simulink model "truck_cabin_sim"  (R2025b)
settings: Solver=FixedStepAuto  StartTime=0.0  StopTime=1000  RelTol=1e-3
values from neighbouring files (symbols this model uses):
  Cth = 50000    [parameters.m]
  HSI_RH_bp = [      0      7.5      17.5      27.5      32.5      37.5      47.5      52.5      72.5      92.5 ]    [HSI_LUT_Setup.m]
  HSI_T_bp = 20:39    [HSI_LUT_Setup.m]
  HSI_Table = 255 * ones(      length(HSI_T_bp),      length(HSI_RH_bp))    [HSI_LUT_Setup.m]
  LowTemp = 20    [HSI_LUT_Setup.m]    (also in hsi_parameters.m = 4)
  Qcool = 3000    [parameters.m]
  RH_initial = 60    [parameters.m]
  T_initial = 25    [parameters.m]
  T_sensor_sigma = 0.2    [parameters.m]
  Ts = 1    [parameters.m]
  UA = 100    [parameters.m]
libraries: simulink x1
settings Model: SnapshotBufferSize=1000  SnapshotInterval=1000  Creator=Admin  LastModifiedBy=Admin
settings OptimizationCC: DefaultParameterBehavior=Inlined  UseDivisionForNetSlopeComputation=on  GainParamInheritBuiltInType=on  UseFloatMulNetSlope=on  InlineInvariantSignals=on  PassReuseOutputArgsAs=Individual arguments  ZeroExternalMemoryAtStartup=off  ZeroInternalMemoryAtStartup=off  NoFixptDivByZeroProtection=on  EfficientFloat2IntCast=on  LifeSpan=1  OptimizeBlockOrder=speed  DifferentSizesBufferReuse=on  EfficientTunableParamExpr=on
settings DebuggingCC: ParameterTunabilityLossMsg=error
settings HardwareCC: ProdLongLongMode=on
settings SFSimCC: MATLABDynamicMemAlloc=off
settings RTWCC: SystemTargetFile=ert.tlc  GenCodeOnly=on  TemplateMakefile=ert_default_tmf  Description=Embedded Coder
settings CodeAppCC: ForceParamTrailComments=on  IgnoreCustomStorageClasses=off  OperatorAnnotations=on  SimulinkDataObjDesc=on  SFDataObjDesc=on  CustomSymbolStrGlobalVar=rt$N$M  CustomSymbolStrType=$N$M  CustomSymbolStrFcn=$N$M$F  CustomSymbolStrMacro=$N$M  InsertBlockDesc=on
settings ERTTargetCC: ERTCustomFileTemplate=example_file_process.tlc  ERTFilePackagingFormat=CompactWithDataFile  TargetLangStandard=C99 (ISO)  GenerateSampleERTMain=on  IncludeMdlTerminateFcn=off  CombineSignalStateStructs=on  SupportComplex=off  SupportContinuousTime=on  SupportNonInlinedSFcns=on

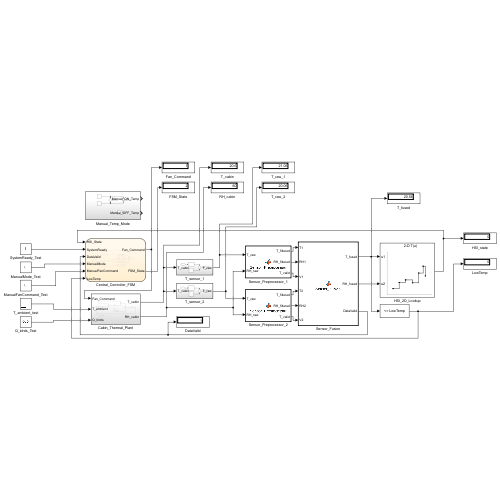
[thumbnail: Simulink's stored preview of the top-level diagram]
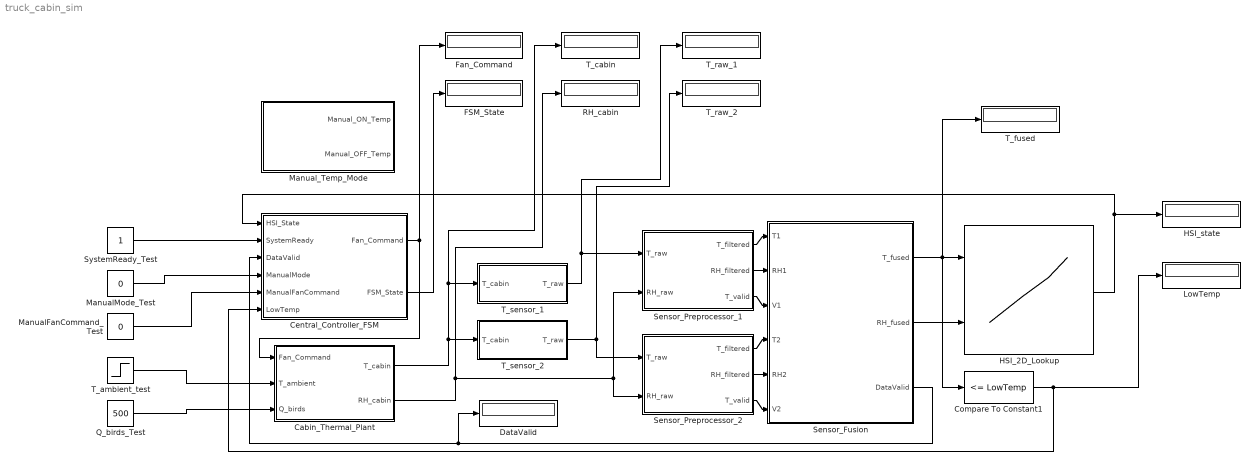
== system truck_cabin_sim ==
  Cabin_Thermal_Plant : Subsystem
  Central_Controller_FSM : Stateflow chart  TreatAsAtomicUnit=on
  Compare To Constant1 : simulink/Logic and Bit Operations/Compare To Constant  relop=<=  const=LowTemp  OutDataTypeStr=boolean
  DataValid : Display
  FSM_State : Display
  Fan_Command : Display
  HSI_2D_Lookup : Lookup_n-D  BreakpointsForDimension1=HSI_T_bp  BreakpointsForDimension2=HSI_RH_bp  Table=HSI_Table  InterpMethod=Flat  InternalRulePriority=Speed  RndMeth=Simplest
      settings: InputPortMap=u0,u1
  HSI_state : Display
  LowTemp : Display
  ManualFanCommand_Test : Constant  Value=0
  ManualMode_Test : Constant  Value=0
  Manual_Temp_Mode : Subsystem
  Q_birds_Test : Constant  Value=500
  RH_cabin : Display
  Sensor_Fusion : MATLAB Function  TreatAsAtomicUnit=on  SystemSampleTime=1
  Sensor_Preprocessor_1 : MATLAB Function  TreatAsAtomicUnit=on  SystemSampleTime=1
  Sensor_Preprocessor_2 : MATLAB Function  TreatAsAtomicUnit=on  SystemSampleTime=1
  SystemReady_Test : Constant
  T_ambient_test : Step  Time=60  Before=20  After=35  SampleTime=Ts
  T_cabin : Display
  T_fused : Display
  T_raw_1 : Display
  T_raw_2 : Display
  T_sensor_1 : Subsystem
  T_sensor_2 : Subsystem
  wires:
  T_ambient_test/1 -> Cabin_Thermal_Plant/2(T_ambient)
  Sensor_Preprocessor_2/2(RH_filtered) -> Sensor_Fusion/5(RH2)
  Sensor_Preprocessor_1/1(T_filtered) -> Sensor_Fusion/1(T1)
  Sensor_Preprocessor_1/2(RH_filtered) -> Sensor_Fusion/2(RH1)
  Sensor_Preprocessor_1/3(T_valid) -> Sensor_Fusion/3(V1)
  Sensor_Preprocessor_2/1(T_filtered) -> Sensor_Fusion/4(T2)
  Sensor_Preprocessor_2/3(T_valid) -> Sensor_Fusion/6(V2)
  Cabin_Thermal_Plant/1(T_cabin) -> T_cabin/1, T_sensor_1/1(T_cabin), T_sensor_2/1(T_cabin)
  T_sensor_1/1(T_raw) -> Sensor_Preprocessor_1/1(T_raw), T_raw_1/1
  T_sensor_2/1(T_raw) -> T_raw_2/1, Sensor_Preprocessor_2/1(T_raw)
  Cabin_Thermal_Plant/2(RH_cabin) -> RH_cabin/1, Sensor_Preprocessor_2/2(RH_raw), Sensor_Preprocessor_1/2(RH_raw)
  Central_Controller_FSM/1(Fan_Command) -> Cabin_Thermal_Plant/1(Fan_Command), Fan_Command/1
  SystemReady_Test/1 -> Central_Controller_FSM/2(SystemReady)
  ManualFanCommand_Test/1 -> Central_Controller_FSM/5(ManualFanCommand)
  ManualMode_Test/1 -> Central_Controller_FSM/4(ManualMode)
  Q_birds_Test/1 -> Cabin_Thermal_Plant/3(Q_birds)
  Central_Controller_FSM/2(FSM_State) -> FSM_State/1
  Sensor_Fusion/3(DataValid) -> Central_Controller_FSM/3(DataValid), DataValid/1
  Sensor_Fusion/2(RH_fused) -> HSI_2D_Lookup/2
  HSI_2D_Lookup/1 -> HSI_state/1, Central_Controller_FSM/1(HSI_State)
  Sensor_Fusion/1(T_fused) -> HSI_2D_Lookup/1, Compare To Constant1/1, T_fused/1
  Compare To Constant1/1 -> LowTemp/1, Central_Controller_FSM/6(LowTemp)

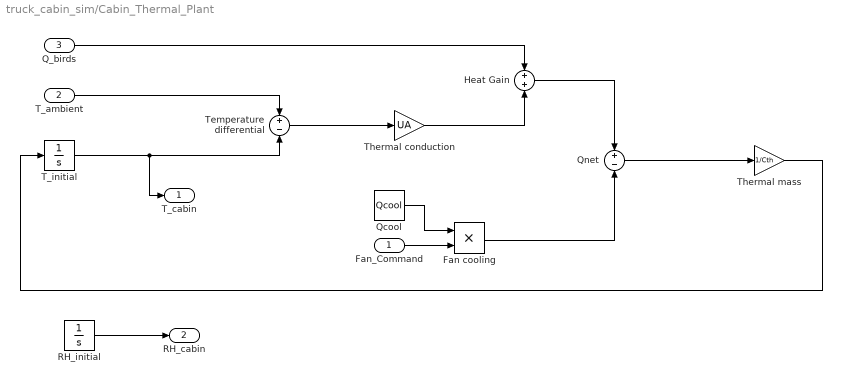
== system truck_cabin_sim/Cabin_Thermal_Plant ==
  Fan_Command : Inport
  T_ambient : Inport  Port=2
  Q_birds : Inport  Port=3
  Fan cooling : Product
  Heat Gain : Sum
  Qcool : Constant  Value=Qcool
  Qnet : Sum  Inputs=+-
  RH_initial : Integrator  InitialCondition=RH_initial
  T_initial : Integrator  InitialCondition=T_initial
  Temperature differential : Sum  Inputs=+-
  Thermal conduction : Gain  Gain=UA
  Thermal mass : Gain  Gain=1/Cth
  T_cabin : Outport
  RH_cabin : Outport  Port=2
  wires:
  T_ambient/1 -> Temperature differential/1
  Temperature differential/1 -> Thermal conduction/1
  Q_birds/1 -> Heat Gain/1
  Thermal conduction/1 -> Heat Gain/2
  Qcool/1 -> Fan cooling/1
  Fan_Command/1 -> Fan cooling/2
  Fan cooling/1 -> Qnet/2
  Heat Gain/1 -> Qnet/1
  Qnet/1 -> Thermal mass/1
  T_initial/1 -> T_cabin/1, Temperature differential/2
  Thermal mass/1 -> T_initial/1
  RH_initial/1 -> RH_cabin/1

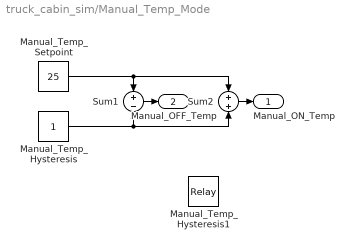
== system truck_cabin_sim/Manual_Temp_Mode ==
  Manual_Temp_Hysteresis : Constant
  Manual_Temp_Hysteresis1 : Relay
  Manual_Temp_Setpoint : Constant  Value=25
  Sum1 : Sum  Inputs=+-
  Sum2 : Sum
  Manual_ON_Temp : Outport
  Manual_OFF_Temp : Outport  Port=2
  wires:
  Manual_Temp_Setpoint/1 -> Sum2/1, Sum1/1
  Manual_Temp_Hysteresis/1 -> Sum2/2, Sum1/2
  Sum2/1 -> Manual_ON_Temp/1
  Sum1/1 -> Manual_OFF_Temp/1

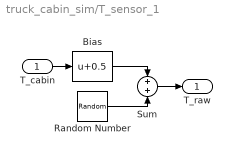
== system truck_cabin_sim/T_sensor_1 ==
  T_cabin : Inport
  Bias : Bias  Bias=0.5  SaturateOnIntegerOverflow=off
  Random Number : RandomNumber  Variance=T_sensor_sigma^2  SampleTime=Ts
  Sum : Sum
  T_raw : Outport
  wires:
  Bias/1 -> Sum/1
  Random Number/1 -> Sum/2
  T_cabin/1 -> Bias/1
  Sum/1 -> T_raw/1

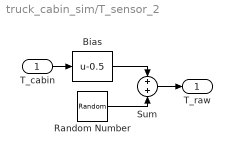
== system truck_cabin_sim/T_sensor_2 ==
  T_cabin : Inport
  Bias : Bias  Bias=-0.5  SaturateOnIntegerOverflow=off
  Random Number : RandomNumber  Variance=T_sensor_sigma^2  SampleTime=Ts
  Sum : Sum
  T_raw : Outport
  wires:
  Bias/1 -> Sum/1
  Random Number/1 -> Sum/2
  T_cabin/1 -> Bias/1
  Sum/1 -> T_raw/1

== matlab function truck_cabin_sim/Sensor_Preprocessor_1 ==
  data: T_raw input; T_filtered output; RH_raw input; RH_filtered output; T_valid output
function [T_filtered, RH_filtered, T_valid] = ...
    Sensor_Preprocessor(T_raw, RH_raw)

persistent T_buffer
persistent RH_buffer
persistent PreviousAcceptedT

if isempty(T_buffer)

    T_buffer = T_raw * ones(1,5);
    RH_buffer = RH_raw * ones(1,5);

    PreviousAcceptedT = T_raw;

end

% ---------------------------------------------------------
% 1. Reject excessive temperature rate
% ---------------------------------------------------------

TempRate = abs(T_raw - PreviousAcceptedT);

if TempRate > 3

    T_valid = false;

    AcceptedT = PreviousAcceptedT;

else

    T_valid = true;

    AcceptedT = T_raw;

    PreviousAcceptedT = T_raw;

end

% ---------------------------------------------------------
% 2. Shift temperature window
% ---------------------------------------------------------

T_buffer(1) = T_buffer(2);
T_buffer(2) = T_buffer(3);
T_buffer(3) = T_buffer(4);
T_buffer(4) = T_buffer(5);
T_buffer(5) = AcceptedT;

% ---------------------------------------------------------
% 3. Shift RH window
% ---------------------------------------------------------

RH_buffer(1) = RH_buffer(2);
RH_buffer(2) = RH_buffer(3);
RH_buffer(3) = RH_buffer(4);
RH_buffer(4) = RH_buffer(5);
RH_buffer(5) = RH_raw;

% ---------------------------------------------------------
% 4. Median
% ---------------------------------------------------------

SortedT = sort(T_buffer);
SortedRH = sort(RH_buffer);

T_filtered = SortedT(3);
RH_filtered = SortedRH(3);

end

== matlab function truck_cabin_sim/Sensor_Preprocessor_2 ==
  data: T_raw input; T_filtered output; RH_raw input; RH_filtered output; T_valid output
function [T_filtered, RH_filtered, T_valid] = ...
    Sensor_Preprocessor(T_raw, RH_raw)

persistent T_buffer
persistent RH_buffer
persistent PreviousAcceptedT

if isempty(T_buffer)

    T_buffer = T_raw * ones(1,5);
    RH_buffer = RH_raw * ones(1,5);

    PreviousAcceptedT = T_raw;

end

% ---------------------------------------------------------
% 1. Reject excessive temperature rate
% ---------------------------------------------------------

TempRate = abs(T_raw - PreviousAcceptedT);

if TempRate > 3

    T_valid = false;

    AcceptedT = PreviousAcceptedT;

else

    T_valid = true;

    AcceptedT = T_raw;

    PreviousAcceptedT = T_raw;

end

% ---------------------------------------------------------
% 2. Shift temperature window
% ---------------------------------------------------------

T_buffer(1) = T_buffer(2);
T_buffer(2) = T_buffer(3);
T_buffer(3) = T_buffer(4);
T_buffer(4) = T_buffer(5);
T_buffer(5) = AcceptedT;

% ---------------------------------------------------------
% 3. Shift RH window
% ---------------------------------------------------------

RH_buffer(1) = RH_buffer(2);
RH_buffer(2) = RH_buffer(3);
RH_buffer(3) = RH_buffer(4);
RH_buffer(4) = RH_buffer(5);
RH_buffer(5) = RH_raw;

% ---------------------------------------------------------
% 4. Median
% ---------------------------------------------------------

SortedT = sort(T_buffer);
SortedRH = sort(RH_buffer);

T_filtered = SortedT(3);
RH_filtered = SortedRH(3);

end

== matlab function truck_cabin_sim/Sensor_Fusion ==
  data: T1 input; T_fused output; RH1 input; V1 input; T2 input; RH2 input; V2 input; RH_fused output; DataValid output
function [T_fused, RH_fused, DataValid] = ...
    Sensor_Fusion(T1, RH1, V1, T2, RH2, V2)

w1 = 0.5;
w2 = 0.5;

sumT = 0;
sumRH = 0;
sumW = 0;

if V1
    sumT = sumT + w1*T1;
    sumRH = sumRH + w1*RH1;
    sumW = sumW + w1;
end

if V2
    sumT = sumT + w2*T2;
    sumRH = sumRH + w2*RH2;
    sumW = sumW + w2;
end

if sumW > 0

    T_fused = sumT / sumW;
    RH_fused = sumRH / sumW;
    DataValid = true;

else

    T_fused = 0;
    RH_fused = 0;
    DataValid = false;

end

== stateflow chart truck_cabin_sim/Central_Controller_FSM ==
  state FAULT
    entry:
    Fan_Command = 0;
    FSM_State = 5;
  state NORMAL
    entry:
    Fan_Command = 0;
    FSM_State = 1;
  state MANUAL
    during:
    Fan_Command = ManualFanCommand;
    FSM_State = 4;
  state INIT
    entry:
    Fan_Command = 0;
    FSM_State = 0;
  state WARNING
    entry:
    Fan_Command = 1;
    FSM_State = 2;
  state CONTROL
    entry:
    Fan_Command = 1;
    FSM_State = 3;
  INIT -> MANUAL [order 5] : [[SystemReady && DataValid && ManualMode]]
  INIT -> FAULT [order 1] : [[~DataValid]]
  CONTROL -> FAULT [order 3] : [[~DataValid]]
  FAULT -> CONTROL [order 3] : [[DataValid && ~ManualMode && HSI_State >= 2]]
  FAULT -> MANUAL [order 4] : [[DataValid && ManualMode]]
  WARNING -> FAULT [order 2] : [[~DataValid]]
  MANUAL -> FAULT [order 4] : [[~DataValid && ~ManualMode]]
  NORMAL -> FAULT [order 3] : [[~DataValid]]
  FAULT -> NORMAL [order 1] : [[DataValid && ~ManualMode && HSI_State == 0]]
  FAULT -> WARNING [order 2] : [[DataValid && ~ManualMode && HSI_State == 1]]
  CONTROL -> NORMAL [order 1] : [HSI_State == 0]
  NORMAL -> MANUAL [order 2] : [[ManualMode]]
  MANUAL -> NORMAL [order 1] : [[~ManualMode && DataValid && HSI_State == 0]]
  WARNING -> MANUAL [order 1] : [[ManualMode]]
  NORMAL -> CONTROL [order 1] : [[HSI_State >= 2]]
  INIT -> NORMAL [order 2] : [[[SystemReady && DataValid && HSI_State == 0]]]
  NORMAL -> WARNING [order 4] : [HSI_State == 1]
  WARNING -> NORMAL [order 4] : [[HSI_State == 0] && LowTemp]
  CONTROL -> MANUAL [order 2] : [[ManualMode]]
  MANUAL -> CONTROL [order 3] : [[~ManualMode && DataValid && HSI_State == 2]]
  MANUAL -> WARNING [order 2] : [[~ManualMode && DataValid && HSI_State == 1]]
  (default) -> INIT
  INIT -> WARNING [order 3] : [[SystemReady && DataValid && HSI_State == 1]]
  INIT -> CONTROL [order 4] : [[SystemReady && DataValid && HSI_State >= 2]]
  WARNING -> CONTROL [order 3] : [[HSI_State >= 2]]
  CONTROL -> WARNING [order 4] : [HSI_State == 1]
  data: HSI_State input; SystemReady input; DataValid input; ManualMode input; ManualFanCommand input; Fan_Command output; FSM_State output; LowTemp input
